simulink model "lab1ex1"  (R2024a)
settings: Solver=VariableStepAuto  StartTime=0.0  StopTime=10.0  RelTol=1e-3

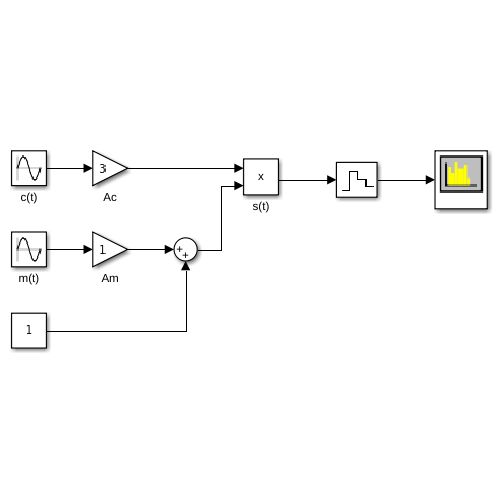
[thumbnail: Simulink's stored preview of the top-level diagram]
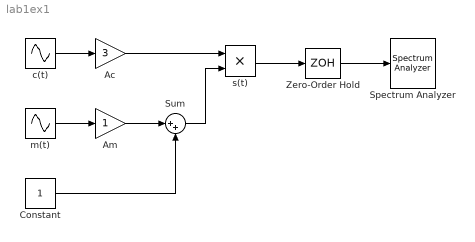
== system lab1ex1 ==
  Ac : Gain  Gain=3
  Am : Gain
  Constant : Constant
  Spectrum Analyzer : SpectrumAnalyzer
  Sum : Sum  Inputs=|++
  Zero-Order Hold : ZeroOrderHold  SampleTime=1/50
  c(t) : Sin  Frequency=2*pi*10  Phase=pi/2  SampleTime=0
  m(t) : Sin  Frequency=2*pi*2  Phase=pi/2  SampleTime=0
  s(t) : Product
  wires:
  Am/1 -> Sum/1
  Constant/1 -> Sum/2
  Sum/1 -> s(t)/2
  Ac/1 -> s(t)/1
  c(t)/1 -> Ac/1
  m(t)/1 -> Am/1
  s(t)/1 -> Zero-Order Hold/1
  Zero-Order Hold/1 -> Spectrum Analyzer/1
